simulink model "simx_tests"  (R2020b)
settings: Solver=VariableStepAuto  StartTime=0.0  StopTime=1  RelTol=1e-3
values from neighbouring files (symbols this model uses):
  CONTROLLER_SAT = 5    [constants.m]
  DAMPING = 0.66784    [constants.m]
  DRIVER_GAIN = 4.8005    [constants.m]
  DRIVER_SAT = 16    [constants.m]
  Kb = 1/22.09592    (= 0.0452572239581)    [constants.m]
  Km = 0.0452    [constants.m]
  SENSOR_GAIN = 1024 / 2*pi    (= 1608.49543864)    [constants.m]
  Wn = 1.3292e7    (= 13292000)    [constants.m]
  ZE_DEN = [L R]    [constants.m]
  ZE_NUM = [1]    [constants.m]
settings Model: Creator=matti  LastModifiedBy=matti

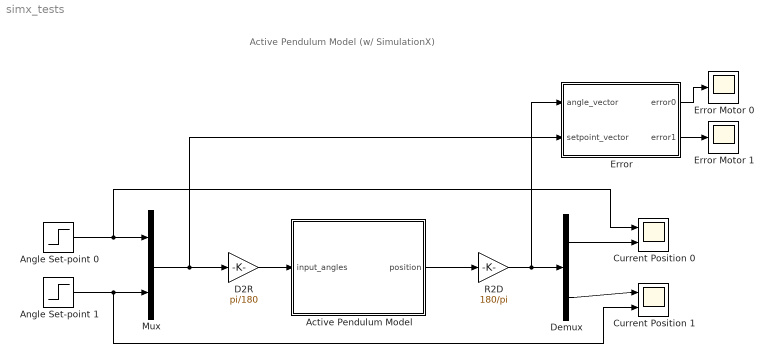
== system simx_tests ==
  note: Active Pendulum Model (w/ SimulationX)
  Active Pendulum Model : Subsystem
  Angle Set-point 0 : Step  Time=0.1  After=90  SampleTime=0
  Angle Set-point 1 : Step  Time=0.1  After=90  SampleTime=0
  Current Position 0 : Scope  NumInputPorts=2
  Current Position 1 : Scope  NumInputPorts=2
  D2R : Gain  Gain=pi/180
  Demux : Demux  Outputs=2
  Error : Subsystem
  Error Motor 0 : Scope
  Error Motor 1 : Scope
  Mux : Mux  Inputs=2
  R2D : Gain  Gain=180/pi
  wires:
  Angle Set-point 0/1 -> Current Position 0/1, Mux/1
  Angle Set-point 1/1 -> Current Position 1/2, Mux/2
  Mux/1 -> Error/2(setpoint_vector), D2R/1
  D2R/1 -> Active Pendulum Model/1(input_angles)
  Active Pendulum Model/1(position) -> R2D/1
  R2D/1 -> Error/1(angle_vector), Demux/1
  Demux/1 -> Current Position 0/2
  Demux/2 -> Current Position 1/1
  Error/1(error0) -> Error Motor 0/1
  Error/2(error1) -> Error Motor 1/1

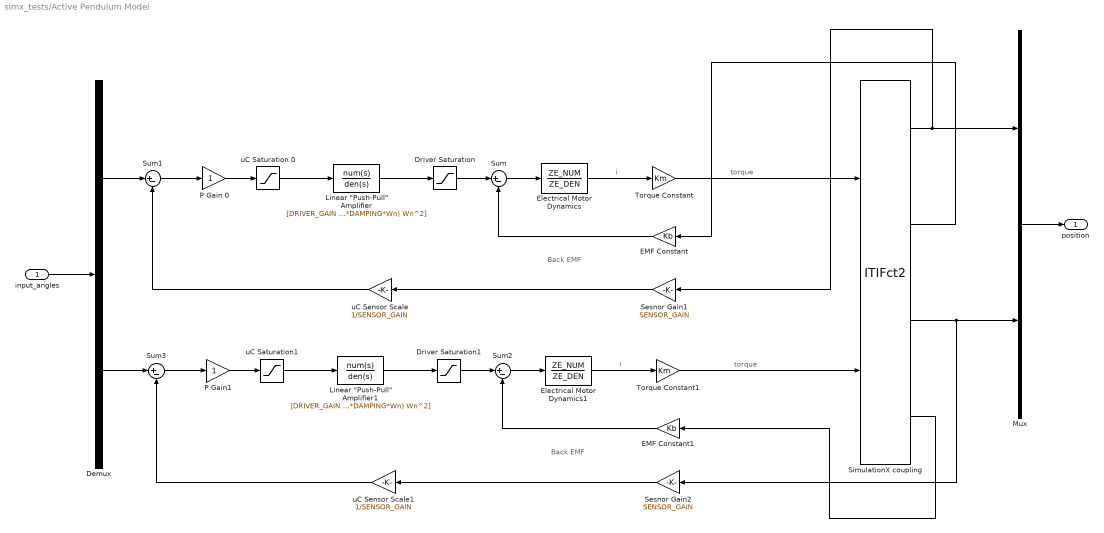
== system simx_tests/Active Pendulum Model ==
  note: Back EMF
  note: torque
  note: i
  note: torque
  note: i
  note: Back EMF
  input_angles : Inport
  Demux : Demux  Outputs=2
  Driver Saturation : Saturate  UpperLimit=DRIVER_SAT  LowerLimit=-DRIVER_SAT
  Driver Saturation1 : Saturate  UpperLimit=DRIVER_SAT  LowerLimit=-DRIVER_SAT
  EMF Constant : Gain  Gain=Kb
  EMF Constant1 : Gain  Gain=Kb
  Electrical Motor Dynamics : TransferFcn  Numerator=ZE_NUM  Denominator=ZE_DEN
  Electrical Motor Dynamics1 : TransferFcn  Numerator=ZE_NUM  Denominator=ZE_DEN
  "Linear \"Push-Pull\" Amplifier" : TransferFcn  Numerator=[DRIVER_GAIN * Wn^2]  Denominator=[1 (2*DAMPING*Wn) Wn^2]
  "Linear \"Push-Pull\" Amplifier1" : TransferFcn  Numerator=[DRIVER_GAIN * Wn^2]  Denominator=[1 (2*DAMPING*Wn) Wn^2]
  Mux : Mux  Inputs=2
  P Gain 0 : Gain
  P Gain1 : Gain
  Sesnor Gain1 : Gain  Gain=SENSOR_GAIN
  Sesnor Gain2 : Gain  Gain=SENSOR_GAIN
  SimulationX coupling : S-Function  FunctionName=ITIFct2  Parameters=ip, port, ts, nIn, nOut  SFunctionDeploymentMode=off  EnableBusSupport=off  mask{ip='localhost', port=4097, ts=0.00001, nIn=2, nOut=4}
      mask prompts: ip "Address: ip"; port "Port Number: port [-]"; ts "Communication Step Size: ts [s]"; nIn "Input Vector Dimension (to SimulationX): nIn [-]"; nOut "Output Vector Dimension (from SimulationX): nOut [-]"
      mask help: Coupling Element
  Sum{,1..3} (4 alike) : Sum  Inputs=|+-
  Torque Constant : Gain  Gain=Km
  Torque Constant1 : Gain  Gain=Km
  uC Saturation 0 : Saturate  UpperLimit=CONTROLLER_SAT  LowerLimit=-CONTROLLER_SAT
  uC Saturation1 : Saturate  UpperLimit=CONTROLLER_SAT  LowerLimit=-CONTROLLER_SAT
  uC Sensor Scale : Gain  Gain=1/SENSOR_GAIN
  uC Sensor Scale1 : Gain  Gain=1/SENSOR_GAIN
  position : Outport
  wires:
  SimulationX coupling/1 -> Sesnor Gain1/1, Mux/1
  uC Sensor Scale/1 -> Sum1/2
  Electrical Motor Dynamics/1 -> Torque Constant/1
  "Linear \"Push-Pull\" Amplifier"/1 -> Driver Saturation/1
  uC Saturation1/1 -> "Linear \"Push-Pull\" Amplifier1"/1
  Driver Saturation/1 -> Sum/1
  Sesnor Gain1/1 -> uC Sensor Scale/1
  SimulationX coupling/2 -> EMF Constant/1
  Sum/1 -> Electrical Motor Dynamics/1
  Sum1/1 -> P Gain 0/1
  uC Saturation 0/1 -> "Linear \"Push-Pull\" Amplifier"/1
  EMF Constant/1 -> Sum/2
  Sum3/1 -> P Gain1/1
  P Gain 0/1 -> uC Saturation 0/1
  Torque Constant1/1 -> SimulationX coupling/2
  EMF Constant1/1 -> Sum2/2
  SimulationX coupling/4 -> EMF Constant1/1
  "Linear \"Push-Pull\" Amplifier1"/1 -> Driver Saturation1/1
  Driver Saturation1/1 -> Sum2/1
  SimulationX coupling/3 -> Mux/2, Sesnor Gain2/1
  uC Sensor Scale1/1 -> Sum3/2
  P Gain1/1 -> uC Saturation1/1
  Sesnor Gain2/1 -> uC Sensor Scale1/1
  Sum2/1 -> Electrical Motor Dynamics1/1
  Torque Constant/1 -> SimulationX coupling/1
  Electrical Motor Dynamics1/1 -> Torque Constant1/1
  Demux/1 -> Sum1/1
  Demux/2 -> Sum3/1
  input_angles/1 -> Demux/1
  Mux/1 -> position/1

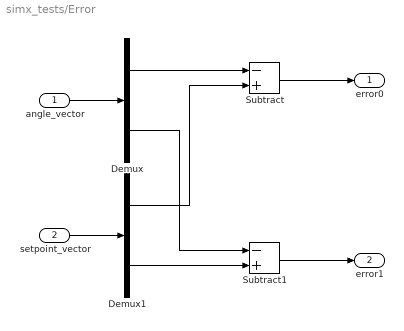
== system simx_tests/Error ==
  angle_vector : Inport
  setpoint_vector : Inport  Port=2
  Demux : Demux  Outputs=2
  Demux1 : Demux  Outputs=2
  Subtract : Sum  Inputs=-+
  Subtract1 : Sum  Inputs=-+
  error0 : Outport
  error1 : Outport  Port=2
  wires:
  Subtract/1 -> error0/1
  angle_vector/1 -> Demux/1
  setpoint_vector/1 -> Demux1/1
  Demux1/1 -> Subtract/2
  Demux/1 -> Subtract/1
  Demux/2 -> Subtract1/1
  Demux1/2 -> Subtract1/2
  Subtract1/1 -> error1/1
